simulink model "RightCameraAgent"  (Simulink 5.0)
settings: Solver=ode45  StartTime=0.0  StopTime=10.0  RelTol=1e-3
settings Model: LastModifiedBy=suarezjl

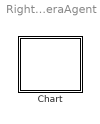
== system RightCameraAgent ==
  Chart : Stateflow chart

== stateflow chart Chart ==
  state Initial
    \\Sally\RightCameraAgent\FrameGrabber.Initialize()
    \\Sally\RightCameraAgent\FrameGrabber.ObtainImage()
    \\Sally\RightCameraAgent\FrameGrabber.ObtainImage()
    \\Sally\RightCameraAgent\ColorSegmenter.Initial()
    \\Sally\RightCameraAgent\ColorSegmenter.LoadColorModel()
  state Segmentation
    \\Sally\RightCameraAgent\FrameGrabber.ObtainImage()
    \\Sally\RightCameraAgent\ColorSegmenter.DoSegment()
  (default) -> Initial : Start
  Initial -> Segmentation : Always
  Segmentation -> Segmentation : Always
